simulink model "mainV02_37"  (R2016b)
settings: Solver=FixedStepAuto  StartTime=0.0  StopTime=inf  FixedStep=Ts  MaxStep=0.2  RelTol=1e-2
undefined symbols (not defined in the file): checks, deltae_degrees, deltafl_degrees, deltafr_degrees, deltar_degrees, deltat_1, deltat_2, deltat_3, deltat_4, deltat_5, Earth, F, ft, groundReaction, initialValues, LD, Light, m, MIL, Newton, Raphson, s, sigbuilder_block, Ts, WGS84
libraries: aerolibutil x19, simulink x17, aerolibtransform2 x7, aerolibasang x4, aerolib6dofsys x4, aerolib6dof2 x4, aerolibwind2 x3, aerolibbdyn x3, aerolibconvert2 x3, aerolibconvert x2, vrlib x2, aerolibatmos2 x1
(part 1 of 5)
settings Model: Creator=Uxío  LastModifiedBy=sork9
settings DataIOCC: ReturnWorkspaceOutputs=on  ReturnWorkspaceOutputsName=spidata
settings OptimizationCC: EfficientMapNaN2IntZero=off  SimCompilerOptimization=on
settings DebuggingCC: ReadBeforeWriteMsg=DisableAll  WriteAfterWriteMsg=DisableAll  WriteAfterReadMsg=DisableAll  MultiTaskDSMMsg=none
settings HardwareCC: TargetBitPerPointer=64  TargetBitPerSizeT=64  TargetBitPerPtrDiffT=64  TargetLongLongMode=on  TargetIntDivRoundTo=Zero  TargetEndianess=LittleEndian  TargetWordSize=64  TargetHWDeviceType=MATLAB Host  ProdEqTarget=off
settings ModelReferenceCC: UpdateModelReferenceTargets=IfOutOfDate
settings SFSimCC: SFSimEcho=off
settings CodeAppCC: MaxIdLength=128
settings GRTTargetCC: TargetLangStandard=C89/C90 (ANSI)  CombineOutputUpdateFcns=off  GRTInterface=on
settings ConfigComp: PSAutoStubLUT=on

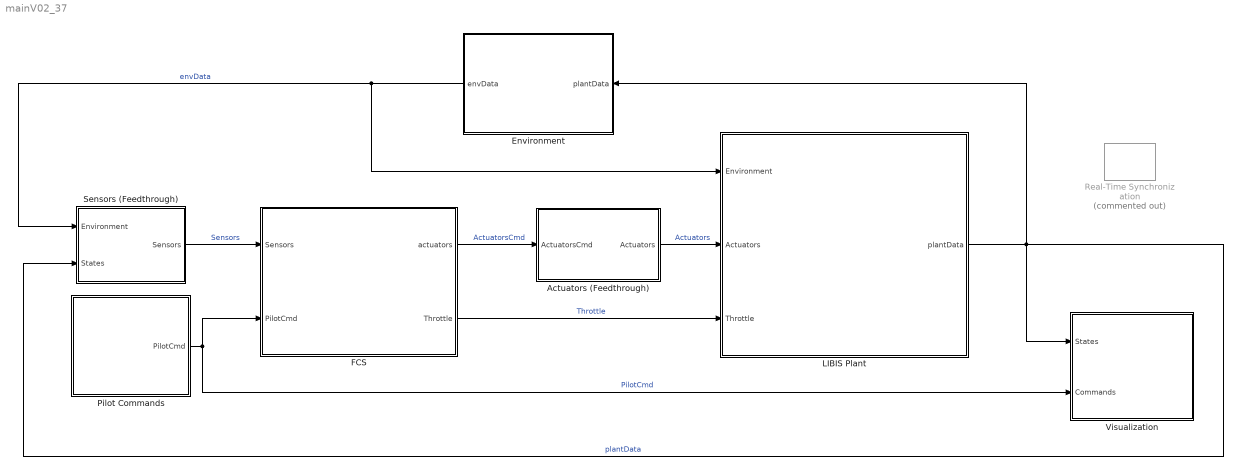
== system mainV02_37 ==
  Actuators (Feedthrough) : Subsystem
  Environment : Subsystem
      mask Display:
      | imageName='Wind.png';
      | currentPath=get_param(bdroot, 'FileName');
      | positions=strfind(currentPath,'\');
      | imagePath=strcat(currentPath(1:positions(end-1)),'graphics\',imageName);
      | image(imagePath);
  FCS : Subsystem
      mask Display:
      | imageName='FCS.png';
      | currentPath=get_param(bdroot, 'FileName');
      | positions=strfind(currentPath,'\');
      | imagePath=strcat(currentPath(1:positions(end-1)),'graphics\',imageName);
      | image(imagePath);
  LIBIS Plant : Subsystem
      mask Display:
      | imageName='LIBIS_Plant.jpg';
      | currentPath=get_param(bdroot, 'FileName');
      | positions=strfind(currentPath,'\');
      | imagePath=strcat(currentPath(1:positions(end-1)),'graphics\',imageName);
      | image(imagePath);
  Pilot Commands : Subsystem  VariantControl=Variants.Command==0
      mask Display:
      | imageName='Pilot.png';
      | currentPath=get_param(bdroot, 'FileName');
      | positions=strfind(currentPath,'\');
      | imagePath=strcat(currentPath(1:positions(end-1)),'graphics\',imageName);
      | image(imagePath);
  Real-Time Synchronization : sldrtlib/Real-Time Synchronization  Commented=on  SampleTime=Ts  MaxMissedTicks=25  ShowMissedTicks=off  YieldWhenWaiting=on
  Sensors (Feedthrough) : Subsystem
  Visualization : Subsystem
  wires:
  FCS/2(Throttle) -> LIBIS Plant/3(Throttle)  "Throttle"
  LIBIS Plant/1(plantData) -> Sensors (Feedthrough)/2(States), Visualization/1(States), Environment/1(plantData)  "plantData"
  Pilot Commands/1(PilotCmd) -> FCS/2(PilotCmd), Visualization/2(Commands)  "PilotCmd"
  Sensors (Feedthrough)/1(Sensors) -> FCS/1(Sensors)  "Sensors"
  Environment/1(envData) -> Sensors (Feedthrough)/1(Environment), LIBIS Plant/1(Environment)  "envData"
  FCS/1(actuators) -> Actuators (Feedthrough)/1(ActuatorsCmd)  "ActuatorsCmd"
  Actuators (Feedthrough)/1(Actuators) -> LIBIS Plant/2(Actuators)  "Actuators"

== system mainV02_37/Actuators (Feedthrough) ==
  ActuatorsCmd : Inport
  Actuators : Outport
  wires:
  ActuatorsCmd/1 -> Actuators/1

== system mainV02_37/Environment ==
  plantData : Inport  OutDataTypeStr=Bus: plantDataBus
  Bus Selector : BusSelector  OutputSignals=LLA.Altitude_m,X_ned,V_ned,Omega_body,CG,DCM_body_earth,LLA.Latitude_deg
  COESA Atmosphere Model : aerolibatmos2/COESA Atmosphere Model  units=Metric (MKS)  spec=1976 COESA-extended U.S. Standard Atmosphere  model=Profile  profile_var=High temperature  profile_percent=1%  profile_alt=5 km (16404 ft)  envelope_var=High temperature  envelope_percent=1%  action=None
  Gravity in Earth Axes : Gain  Gain=[0 0 LD.Inertia.mass]  SaturateOnIntegerOverflow=on  OutDataTypeStr=Inherit: Same as input  ParamDataTypeStr=Inherit: Same as input
  IC : InitialCondition  Value=[0 0 0]
  Math Function : Math  Operator=transpose  SaturateOnIntegerOverflow=on
  Reshape : Reshape
  Reshape1 : Reshape
  Reshape2 : Reshape
  Terrain : Subsystem
  To Body Axes : Product  Multiplication=Matrix(*)  SaturateOnIntegerOverflow=on  InputSameDT=on  OutDataTypeStr=Inherit: Same as first input
  WGS84 Gravity Model : aerolibobsolete/WGS84 Gravity Model  model=WGS84 Taylor Series  units=Metric (MKS)  no_atmos=on  precessing=on  month=February  day=1  year=2000  no_centrifugal=on  action=None
  Wind Models : Subsystem
  envDataBus : BusCreator  Inputs='h_ground','Fground','Mground','windVelocity','windOmega','T','a','P','AirDensity','Fgravity'  OutDataTypeStr=Bus: envDataBus  NonVirtualBus=on
  envData : Outport  OutDataTypeStr=Bus: envDataBus  InitialOutput=0
  wires:
  [Altitude] -> COESA Atmosphere Model/1
  Bus Selector/6 -> To Body Axes/1, Wind Models/3(DCM_be), Terrain/4(DCM_body_earth)  "<DCM_body_earth>"
  Bus Selector/7 -> WGS84 Gravity Model/2  "<Latitude_deg>"
  Bus Selector/3 -> Terrain/2(Ve), Wind Models/1(Ve)  "<V_ned>"
  [Altitude] -> WGS84 Gravity Model/1
  envDataBus/1 -> envData/1  "envData"
  To Body Axes/1 -> Reshape/1  "Fg"
  Wind Models/2(windOmega) -> envDataBus/5  "windOmega"
  Bus Selector/2 -> Terrain/1(Xe)  "<X_ned>"
  WGS84 Gravity Model/1 -> Gravity in Earth Axes/1
  COESA Atmosphere Model/3 -> envDataBus/8  "P"
  COESA Atmosphere Model/2 -> envDataBus/7  "a"
  Wind Models/1(windVelocity) -> envDataBus/4  "windVelocity"
  [Altitude] -> Wind Models/2(Altitude)
  COESA Atmosphere Model/1 -> envDataBus/6  "T"
  COESA Atmosphere Model/4 -> envDataBus/9  "AirDensity"
  Terrain/1(hground) -> envDataBus/1  "h_ground"
  Bus Selector/1 -> [Altitude]  "<Altitude_m>"
  Gravity in Earth Axes/1 -> Math Function/1
  Math Function/1 -> To Body Axes/2
  Reshape/1 -> envDataBus/10  "Fgravity"
  Reshape1/1 -> envDataBus/2  "Fground"
  plantData/1 -> Bus Selector/1
  Bus Selector/5 -> Terrain/5("CG ")  "<CG>"
  Reshape2/1 -> envDataBus/3  "Mground"
  Bus Selector/4 -> Terrain/3("Omega_body ")  "<Omega_body>"
  Terrain/2(Fground) -> IC/1
  Terrain/3(Mground) -> Reshape2/1
  IC/1 -> Reshape1/1

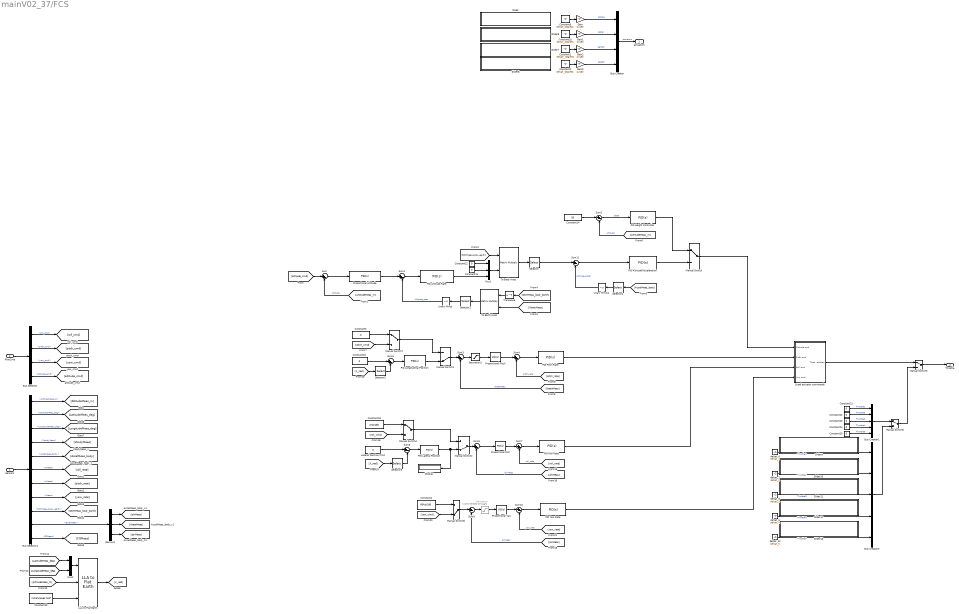
== system mainV02_37/FCS ==
  Sensors : Inport  OutDataTypeStr=Bus: SensorsBus
  PilotCmd : Inport  Port=2  OutDataTypeStr=Bus: CommandBus
  Bus Creator : BusCreator  Inputs=4
  Bus Creator1 : BusCreator  Inputs=5  OutDataTypeStr=Bus: ThrottleBus
  Bus Creator3 : BusCreator  Inputs=5
  Bus Selector : BusSelector  OutputSignals=roll_cmd,pitch_cmd,yaw_cmd,altitude_cmd
  Bus Selector1 : BusSelector  OutputSignals=LLAMeas.AltitudeMeas_m,LLAMeas.LatitudeMeas_deg,LLAMeas.LongitudeMeas_deg,VbodyMeas,AccelMeas_body,OmegaMeas_body.pMeas,OmegaMeas_body.qMeas,OmegaMeas_body.rMeas,DCMMeas_body_earth,EulerMeas,CGMeas
  Constant1 : Constant  Value=deltafr_degrees
  Constant10 : Constant  Value=deltar_degrees
  Constant{3,11..12,16,20..24} (9 alike) : Constant  Value=0
  Constant13 : Constant  Value=initialValues.href
  Constant14 : Constant  Value=50
  Constant18 : Constant  Value=2*pi/180
  Constant2 : Constant  Value=deltafl_degrees
  Constant4 : Constant  Value=60*pi/180
  Constant9 : Constant  Value=deltae_degrees
  Demux3 : Demux  Outputs=3
  Display : Display
  Gain{,1..3} (4 alike) : Gain  Gain=pi/180
  LLA to Flat Earth : aerolibtransform2/LLA to Flat Earth  units=Metric (MKS)  ptype=Earth (WGS84)  F=1/298.257223563  R=6378137  LL0=initialValues.LatLong0  psi=0
  Lateral Position Cmd : Constant  Value=0
  Manual Switch{,3..5,7} (5 alike) : ManualSwitch
  Manual Switch1 : ManualSwitch  CurrentSetting=0
  Manual Switch2 : ManualSwitch  CurrentSetting=0
  Manual Switch6 : ManualSwitch  CurrentSetting=0
  Mux1 : Mux  Inputs=3
  Mux2 : Mux  Inputs=2
  PID Altitude Acceleration : simulink/Continuous/PID Controller  Controller=PID  TimeDomain=Continuous-time  SampleTime=-1  IntegratorMethod=Forward Euler  FilterMethod=Forward Euler  Form=Parallel  UseFilter=on  ControllerParametersSource=internal  P=1  I=1  D=0  N=100  InitialConditionSource=internal  InitialConditionForIntegrator=0  InitialConditionForFilter=0  ExternalReset=none  LimitOutput=on  UpperSaturationLimit=1.5*9.81  LowerSaturationLimit=0.5*9.81  LinearizeAsGain=on  AntiWindupMode=none  Kb=1  TrackingMode=off  Kt=1  PParamMin=[]  PParamMax=[]  IParamMin=[]  IParamMax=[]  DParamMin=[]  DParamMax=[]  NParamMin=[]  NParamMax=[]  KbParamMin=[]  KbParamMax=[]  KtParamMin=[]  KtParamMax=[]  POutMin=[]  POutMax=[]  IOutMin=[]  IOutMax=[]  DOutMin=[]  DOutMax=[]  NOutMin=[]  NOutMax=[]  KbOutMin=[]  KbOutMax=[]  KtOutMin=[]  KtOutMax=[]  IntegratorOutMin=[]  IntegratorOutMax=[]  FilterOutMin=[]  FilterOutMax=[]  SumOutMin=[]  SumOutMax=[]  SumI1OutMin=[]  SumI1OutMax=[]  SumI2OutMin=[]  SumI2OutMax=[]  SumI3OutMin=[]  SumI3OutMax=[]  SumDOutMin=[]  SumDOutMax=[]  SaturationOutMin=[]  SaturationOutMax=[]  IntegratorContinuousStateAttributes=''  IntegratorStateMustResolveToSignalObject=off  IntegratorRTWStateStorageClass=Auto  FilterContinuousStateAttributes=''  FilterStateMustResolveToSignalObject=off  FilterRTWStateStorageClass=Auto  DifferentiatorICPrevScaledInput=0  DifferentiatorOutMin=[]  DifferentiatorOutMax=[]
  PID Altitude Rate : simulink/Continuous/PID Controller  Controller=PID  TimeDomain=Continuous-time  SampleTime=-1  IntegratorMethod=Forward Euler  FilterMethod=Forward Euler  Form=Parallel  UseFilter=on  ControllerParametersSource=internal  P=1  I=1  D=0  N=100  InitialConditionSource=internal  InitialConditionForIntegrator=0  InitialConditionForFilter=0  ExternalReset=none  LimitOutput=on  UpperSaturationLimit=1.5*9.81  LowerSaturationLimit=0.5*9.81  LinearizeAsGain=on  AntiWindupMode=none  Kb=1  TrackingMode=off  Kt=1  PParamMin=[]  PParamMax=[]  IParamMin=[]  IParamMax=[]  DParamMin=[]  DParamMax=[]  NParamMin=[]  NParamMax=[]  KbParamMin=[]  KbParamMax=[]  KtParamMin=[]  KtParamMax=[]  POutMin=[]  POutMax=[]  IOutMin=[]  IOutMax=[]  DOutMin=[]  DOutMax=[]  NOutMin=[]  NOutMax=[]  KbOutMin=[]  KbOutMax=[]  KtOutMin=[]  KtOutMax=[]  IntegratorOutMin=[]  IntegratorOutMax=[]  FilterOutMin=[]  FilterOutMax=[]  SumOutMin=[]  SumOutMax=[]  SumI1OutMin=[]  SumI1OutMax=[]  SumI2OutMin=[]  SumI2OutMax=[]  SumI3OutMin=[]  SumI3OutMax=[]  SumDOutMin=[]  SumDOutMax=[]  SaturationOutMin=[]  SaturationOutMax=[]  IntegratorContinuousStateAttributes=''  IntegratorStateMustResolveToSignalObject=off  IntegratorRTWStateStorageClass=Auto  FilterContinuousStateAttributes=''  FilterStateMustResolveToSignalObject=off  FilterRTWStateStorageClass=Auto  DifferentiatorICPrevScaledInput=0  DifferentiatorOutMin=[]  DifferentiatorOutMax=[]
  PID Height Controller : simulink/Continuous/PID Controller  Controller=PID  TimeDomain=Continuous-time  SampleTime=-1  IntegratorMethod=Forward Euler  FilterMethod=Forward Euler  Form=Parallel  UseFilter=on  ControllerParametersSource=internal  P=0.5  I=0.25  D=0.5  N=100  InitialConditionSource=internal  InitialConditionForIntegrator=0  InitialConditionForFilter=0  ExternalReset=none  LimitOutput=on  UpperSaturationLimit=1  LowerSaturationLimit=0  LinearizeAsGain=on  AntiWindupMode=clamping  Kb=1  TrackingMode=off  Kt=1  PParamMin=[]  PParamMax=[]  IParamMin=[]  IParamMax=[]  DParamMin=[]  DParamMax=[]  NParamMin=[]  NParamMax=[]  KbParamMin=[]  KbParamMax=[]  KtParamMin=[]  KtParamMax=[]  POutMin=[]  POutMax=[]  IOutMin=[]  IOutMax=[]  DOutMin=[]  DOutMax=[]  NOutMin=[]  NOutMax=[]  KbOutMin=[]  KbOutMax=[]  KtOutMin=[]  KtOutMax=[]  IntegratorOutMin=[]  IntegratorOutMax=[]  FilterOutMin=[]  FilterOutMax=[]  SumOutMin=[]  SumOutMax=[]  SumI1OutMin=[]  SumI1OutMax=[]  SumI2OutMin=[]  SumI2OutMax=[]  SumI3OutMin=[]  SumI3OutMax=[]  SumDOutMin=[]  SumDOutMax=[]  SaturationOutMin=[]  SaturationOutMax=[]  IntegratorContinuousStateAttributes=''  IntegratorStateMustResolveToSignalObject=off  IntegratorRTWStateStorageClass=Auto  FilterContinuousStateAttributes=''  FilterStateMustResolveToSignalObject=off  FilterRTWStateStorageClass=Auto  DifferentiatorICPrevScaledInput=0  DifferentiatorOutMin=[]  DifferentiatorOutMax=[]
  PID Lateral Position : simulink/Continuous/PID Controller  Controller=PID  TimeDomain=Continuous-time  SampleTime=-1  IntegratorMethod=Forward Euler  FilterMethod=Forward Euler  Form=Parallel  UseFilter=on  ControllerParametersSource=internal  P=0.1  I=0  D=0.3  N=100  InitialConditionSource=internal  InitialConditionForIntegrator=0  InitialConditionForFilter=0  ExternalReset=none  LimitOutput=on  UpperSaturationLimit=30*pi/180  LowerSaturationLimit=-30*pi/180  LinearizeAsGain=on  AntiWindupMode=none  Kb=1  TrackingMode=off  Kt=1  PParamMin=[]  PParamMax=[]  IParamMin=[]  IParamMax=[]  DParamMin=[]  DParamMax=[]  NParamMin=[]  NParamMax=[]  KbParamMin=[]  KbParamMax=[]  KtParamMin=[]  KtParamMax=[]  POutMin=[]  POutMax=[]  IOutMin=[]  IOutMax=[]  DOutMin=[]  DOutMax=[]  NOutMin=[]  NOutMax=[]  KbOutMin=[]  KbOutMax=[]  KtOutMin=[]  KtOutMax=[]  IntegratorOutMin=[]  IntegratorOutMax=[]  FilterOutMin=[]  FilterOutMax=[]  SumOutMin=[]  SumOutMax=[]  SumI1OutMin=[]  SumI1OutMax=[]  SumI2OutMin=[]  SumI2OutMax=[]  SumI3OutMin=[]  SumI3OutMax=[]  SumDOutMin=[]  SumDOutMax=[]  SaturationOutMin=[]  SaturationOutMax=[]  IntegratorContinuousStateAttributes=''  IntegratorStateMustResolveToSignalObject=off  IntegratorRTWStateStorageClass=Auto  FilterContinuousStateAttributes=''  FilterStateMustResolveToSignalObject=off  FilterRTWStateStorageClass=Auto  DifferentiatorICPrevScaledInput=0  DifferentiatorOutMin=[]  DifferentiatorOutMax=[]
  PID Longitudinal Position : simulink/Continuous/PID Controller  Controller=PID  TimeDomain=Continuous-time  SampleTime=-1  IntegratorMethod=Forward Euler  FilterMethod=Forward Euler  Form=Parallel  UseFilter=on  ControllerParametersSource=internal  P=-0.1  I=0  D=-0.3  N=100  InitialConditionSource=internal  InitialConditionForIntegrator=0  InitialConditionForFilter=0  ExternalReset=none  LimitOutput=on  UpperSaturationLimit=30*pi/180  LowerSaturationLimit=-30*pi/180  LinearizeAsGain=on  AntiWindupMode=none  Kb=1  TrackingMode=off  Kt=1  PParamMin=[]  PParamMax=[]  IParamMin=[]  IParamMax=[]  DParamMin=[]  DParamMax=[]  NParamMin=[]  NParamMax=[]  KbParamMin=[]  KbParamMax=[]  KtParamMin=[]  KtParamMax=[]  POutMin=[]  POutMax=[]  IOutMin=[]  IOutMax=[]  DOutMin=[]  DOutMax=[]  NOutMin=[]  NOutMax=[]  KbOutMin=[]  KbOutMax=[]  KtOutMin=[]  KtOutMax=[]  IntegratorOutMin=[]  IntegratorOutMax=[]  FilterOutMin=[]  FilterOutMax=[]  SumOutMin=[]  SumOutMax=[]  SumI1OutMin=[]  SumI1OutMax=[]  SumI2OutMin=[]  SumI2OutMax=[]  SumI3OutMin=[]  SumI3OutMax=[]  SumDOutMin=[]  SumDOutMax=[]  SaturationOutMin=[]  SaturationOutMax=[]  IntegratorContinuousStateAttributes=''  IntegratorStateMustResolveToSignalObject=off  IntegratorRTWStateStorageClass=Auto  FilterContinuousStateAttributes=''  FilterStateMustResolveToSignalObject=off  FilterRTWStateStorageClass=Auto  DifferentiatorICPrevScaledInput=0  DifferentiatorOutMin=[]  DifferentiatorOutMax=[]
  PID Pitch Rate : simulink/Continuous/PID Controller  Controller=PID  TimeDomain=Continuous-time  SampleTime=-1  IntegratorMethod=Forward Euler  FilterMethod=Forward Euler  Form=Parallel  UseFilter=on  ControllerParametersSource=internal  P=2  I=1  D=0  N=100  InitialConditionSource=internal  InitialConditionForIntegrator=0  InitialConditionForFilter=0  ExternalReset=none  LimitOutput=on  UpperSaturationLimit=0.5  LowerSaturationLimit=-0.5  LinearizeAsGain=on  AntiWindupMode=none  Kb=1  TrackingMode=off  Kt=1  PParamMin=[]  PParamMax=[]  IParamMin=[]  IParamMax=[]  DParamMin=[]  DParamMax=[]  NParamMin=[]  NParamMax=[]  KbParamMin=[]  KbParamMax=[]  KtParamMin=[]  KtParamMax=[]  POutMin=[]  POutMax=[]  IOutMin=[]  IOutMax=[]  DOutMin=[]  DOutMax=[]  NOutMin=[]  NOutMax=[]  KbOutMin=[]  KbOutMax=[]  KtOutMin=[]  KtOutMax=[]  IntegratorOutMin=[]  IntegratorOutMax=[]  FilterOutMin=[]  FilterOutMax=[]  SumOutMin=[]  SumOutMax=[]  SumI1OutMin=[]  SumI1OutMax=[]  SumI2OutMin=[]  SumI2OutMax=[]  SumI3OutMin=[]  SumI3OutMax=[]  SumDOutMin=[]  SumDOutMax=[]  SaturationOutMin=[]  SaturationOutMax=[]  IntegratorContinuousStateAttributes=''  IntegratorStateMustResolveToSignalObject=off  IntegratorRTWStateStorageClass=Auto  FilterContinuousStateAttributes=''  FilterStateMustResolveToSignalObject=off  FilterRTWStateStorageClass=Auto  DifferentiatorICPrevScaledInput=0  DifferentiatorOutMin=[]  DifferentiatorOutMax=[]
  PID Roll Rate : simulink/Continuous/PID Controller  Controller=PID  TimeDomain=Continuous-time  SampleTime=-1  IntegratorMethod=Forward Euler  FilterMethod=Forward Euler  Form=Parallel  UseFilter=on  ControllerParametersSource=internal  P=4  I=0  D=0  N=100  InitialConditionSource=internal  InitialConditionForIntegrator=0  InitialConditionForFilter=0  ExternalReset=none  LimitOutput=on  UpperSaturationLimit=0.5  LowerSaturationLimit=-0.5  LinearizeAsGain=on  AntiWindupMode=none  Kb=1  TrackingMode=off  Kt=1  PParamMin=[]  PParamMax=[]  IParamMin=[]  IParamMax=[]  DParamMin=[]  DParamMax=[]  NParamMin=[]  NParamMax=[]  KbParamMin=[]  KbParamMax=[]  KtParamMin=[]  KtParamMax=[]  POutMin=[]  POutMax=[]  IOutMin=[]  IOutMax=[]  DOutMin=[]  DOutMax=[]  NOutMin=[]  NOutMax=[]  KbOutMin=[]  KbOutMax=[]  KtOutMin=[]  KtOutMax=[]  IntegratorOutMin=[]  IntegratorOutMax=[]  FilterOutMin=[]  FilterOutMax=[]  SumOutMin=[]  SumOutMax=[]  SumI1OutMin=[]  SumI1OutMax=[]  SumI2OutMin=[]  SumI2OutMax=[]  SumI3OutMin=[]  SumI3OutMax=[]  SumDOutMin=[]  SumDOutMax=[]  SaturationOutMin=[]  SaturationOutMax=[]  IntegratorContinuousStateAttributes=''  IntegratorStateMustResolveToSignalObject=off  IntegratorRTWStateStorageClass=Auto  FilterContinuousStateAttributes=''  FilterStateMustResolveToSignalObject=off  FilterRTWStateStorageClass=Auto  DifferentiatorICPrevScaledInput=0  DifferentiatorOutMin=[]  DifferentiatorOutMax=[]
  PID Yaw Rate : simulink/Continuous/PID Controller  Controller=PID  TimeDomain=Continuous-time  SampleTime=-1  IntegratorMethod=Forward Euler  FilterMethod=Forward Euler  Form=Parallel  UseFilter=on  ControllerParametersSource=internal  P=5  I=0  D=0  N=100  InitialConditionSource=internal  InitialConditionForIntegrator=0  InitialConditionForFilter=0  ExternalReset=none  LimitOutput=on  UpperSaturationLimit=0.1  LowerSaturationLimit=-0.1  LinearizeAsGain=on  AntiWindupMode=none  Kb=1  TrackingMode=off  Kt=1  PParamMin=[]  PParamMax=[]  IParamMin=[]  IParamMax=[]  DParamMin=[]  DParamMax=[]  NParamMin=[]  NParamMax=[]  KbParamMin=[]  KbParamMax=[]  KtParamMin=[]  KtParamMax=[]  POutMin=[]  POutMax=[]  IOutMin=[]  IOutMax=[]  DOutMin=[]  DOutMax=[]  NOutMin=[]  NOutMax=[]  KbOutMin=[]  KbOutMax=[]  KtOutMin=[]  KtOutMax=[]  IntegratorOutMin=[]  IntegratorOutMax=[]  FilterOutMin=[]  FilterOutMax=[]  SumOutMin=[]  SumOutMax=[]  SumI1OutMin=[]  SumI1OutMax=[]  SumI2OutMin=[]  SumI2OutMax=[]  SumI3OutMin=[]  SumI3OutMax=[]  SumDOutMin=[]  SumDOutMax=[]  SaturationOutMin=[]  SaturationOutMax=[]  IntegratorContinuousStateAttributes=''  IntegratorStateMustResolveToSignalObject=off  IntegratorRTWStateStorageClass=Auto  FilterContinuousStateAttributes=''  FilterStateMustResolveToSignalObject=off  FilterRTWStateStorageClass=Auto  DifferentiatorICPrevScaledInput=0  DifferentiatorOutMin=[]  DifferentiatorOutMax=[]
  Proportional Altitude : simulink/Continuous/PID Controller  Controller=PID  TimeDomain=Continuous-time  SampleTime=-1  IntegratorMethod=Forward Euler  FilterMethod=Forward Euler  Form=Parallel  UseFilter=on  ControllerParametersSource=internal  P=-1  I=0  D=0  N=100  InitialConditionSource=internal  InitialConditionForIntegrator=0  InitialConditionForFilter=0  ExternalReset=none  LimitOutput=on  UpperSaturationLimit=250  LowerSaturationLimit=-inf  LinearizeAsGain=on  AntiWindupMode=none  Kb=1  TrackingMode=off  Kt=1  PParamMin=[]  PParamMax=[]  IParamMin=[]  IParamMax=[]  DParamMin=[]  DParamMax=[]  NParamMin=[]  NParamMax=[]  KbParamMin=[]  KbParamMax=[]  KtParamMin=[]  KtParamMax=[]  POutMin=[]  POutMax=[]  IOutMin=[]  IOutMax=[]  DOutMin=[]  DOutMax=[]  NOutMin=[]  NOutMax=[]  KbOutMin=[]  KbOutMax=[]  KtOutMin=[]  KtOutMax=[]  IntegratorOutMin=[]  IntegratorOutMax=[]  FilterOutMin=[]  FilterOutMax=[]  SumOutMin=[]  SumOutMax=[]  SumI1OutMin=[]  SumI1OutMax=[]  SumI2OutMin=[]  SumI2OutMax=[]  SumI3OutMin=[]  SumI3OutMax=[]  SumDOutMin=[]  SumDOutMax=[]  SaturationOutMin=[]  SaturationOutMax=[]  IntegratorContinuousStateAttributes=''  IntegratorStateMustResolveToSignalObject=off  IntegratorRTWStateStorageClass=Auto  FilterContinuousStateAttributes=''  FilterStateMustResolveToSignalObject=off  FilterRTWStateStorageClass=Auto  DifferentiatorICPrevScaledInput=0  DifferentiatorOutMin=[]  DifferentiatorOutMax=[]
  Proportional Pitch : simulink/Continuous/PID Controller  Controller=PID  TimeDomain=Continuous-time  SampleTime=-1  IntegratorMethod=Forward Euler  FilterMethod=Forward Euler  Form=Parallel  UseFilter=on  ControllerParametersSource=internal  P=4  I=0  D=0  N=100  InitialConditionSource=internal  InitialConditionForIntegrator=0  InitialConditionForFilter=0  ExternalReset=none  LimitOutput=off  UpperSaturationLimit=inf  LowerSaturationLimit=-inf  LinearizeAsGain=on  AntiWindupMode=none  Kb=1  TrackingMode=off  Kt=1  PParamMin=[]  PParamMax=[]  IParamMin=[]  IParamMax=[]  DParamMin=[]  DParamMax=[]  NParamMin=[]  NParamMax=[]  KbParamMin=[]  KbParamMax=[]  KtParamMin=[]  KtParamMax=[]  POutMin=[]  POutMax=[]  IOutMin=[]  IOutMax=[]  DOutMin=[]  DOutMax=[]  NOutMin=[]  NOutMax=[]  KbOutMin=[]  KbOutMax=[]  KtOutMin=[]  KtOutMax=[]  IntegratorOutMin=[]  IntegratorOutMax=[]  FilterOutMin=[]  FilterOutMax=[]  SumOutMin=[]  SumOutMax=[]  SumI1OutMin=[]  SumI1OutMax=[]  SumI2OutMin=[]  SumI2OutMax=[]  SumI3OutMin=[]  SumI3OutMax=[]  SumDOutMin=[]  SumDOutMax=[]  SaturationOutMin=[]  SaturationOutMax=[]  IntegratorContinuousStateAttributes=''  IntegratorStateMustResolveToSignalObject=off  IntegratorRTWStateStorageClass=Auto  FilterContinuousStateAttributes=''  FilterStateMustResolveToSignalObject=off  FilterRTWStateStorageClass=Auto  DifferentiatorICPrevScaledInput=0  DifferentiatorOutMin=[]  DifferentiatorOutMax=[]
  Proportional Roll : simulink/Continuous/PID Controller  Controller=PID  TimeDomain=Continuous-time  SampleTime=-1  IntegratorMethod=Forward Euler  FilterMethod=Forward Euler  Form=Parallel  UseFilter=on  ControllerParametersSource=internal  P=1  I=0  D=0  N=100  InitialConditionSource=internal  InitialConditionForIntegrator=0  InitialConditionForFilter=0  ExternalReset=none  LimitOutput=off  UpperSaturationLimit=inf  LowerSaturationLimit=-inf  LinearizeAsGain=on  AntiWindupMode=none  Kb=1  TrackingMode=off  Kt=1  PParamMin=[]  PParamMax=[]  IParamMin=[]  IParamMax=[]  DParamMin=[]  DParamMax=[]  NParamMin=[]  NParamMax=[]  KbParamMin=[]  KbParamMax=[]  KtParamMin=[]  KtParamMax=[]  POutMin=[]  POutMax=[]  IOutMin=[]  IOutMax=[]  DOutMin=[]  DOutMax=[]  NOutMin=[]  NOutMax=[]  KbOutMin=[]  KbOutMax=[]  KtOutMin=[]  KtOutMax=[]  IntegratorOutMin=[]  IntegratorOutMax=[]  FilterOutMin=[]  FilterOutMax=[]  SumOutMin=[]  SumOutMax=[]  SumI1OutMin=[]  SumI1OutMax=[]  SumI2OutMin=[]  SumI2OutMax=[]  SumI3OutMin=[]  SumI3OutMax=[]  SumDOutMin=[]  SumDOutMax=[]  SaturationOutMin=[]  SaturationOutMax=[]  IntegratorContinuousStateAttributes=''  IntegratorStateMustResolveToSignalObject=off  IntegratorRTWStateStorageClass=Auto  FilterContinuousStateAttributes=''  FilterStateMustResolveToSignalObject=off  FilterRTWStateStorageClass=Auto  DifferentiatorICPrevScaledInput=0  DifferentiatorOutMin=[]  DifferentiatorOutMax=[]
  Proportional Yaw : simulink/Continuous/PID Controller  Controller=PID  TimeDomain=Continuous-time  SampleTime=-1  IntegratorMethod=Forward Euler  FilterMethod=Forward Euler  Form=Parallel  UseFilter=on  ControllerParametersSource=internal  P=1  I=0  D=0  N=100  InitialConditionSource=internal  InitialConditionForIntegrator=0  InitialConditionForFilter=0  ExternalReset=none  LimitOutput=off  UpperSaturationLimit=30*pi/180  LowerSaturationLimit=-30*pi/180  LinearizeAsGain=on  AntiWindupMode=none  Kb=1  TrackingMode=off  Kt=1  PParamMin=[]  PParamMax=[]  IParamMin=[]  IParamMax=[]  DParamMin=[]  DParamMax=[]  NParamMin=[]  NParamMax=[]  KbParamMin=[]  KbParamMax=[]  KtParamMin=[]  KtParamMax=[]  POutMin=[]  POutMax=[]  IOutMin=[]  IOutMax=[]  DOutMin=[]  DOutMax=[]  NOutMin=[]  NOutMax=[]  KbOutMin=[]  KbOutMax=[]  KtOutMin=[]  KtOutMax=[]  IntegratorOutMin=[]  IntegratorOutMax=[]  FilterOutMin=[]  FilterOutMax=[]  SumOutMin=[]  SumOutMax=[]  SumI1OutMin=[]  SumI1OutMax=[]  SumI2OutMin=[]  SumI2OutMax=[]  SumI3OutMin=[]  SumI3OutMax=[]  SumDOutMin=[]  SumDOutMax=[]  SaturationOutMin=[]  SaturationOutMax=[]  IntegratorContinuousStateAttributes=''  IntegratorStateMustResolveToSignalObject=off  IntegratorRTWStateStorageClass=Auto  FilterContinuousStateAttributes=''  FilterStateMustResolveToSignalObject=off  FilterRTWStateStorageClass=Auto  DifferentiatorICPrevScaledInput=0  DifferentiatorOutMin=[]  DifferentiatorOutMax=[]
  Quad actuator commands : Subsystem
  Saturation : Saturate  Commented=through  UpperLimit=30*pi/180  LowerLimit=-30*pi/180
  Saturation1 : Saturate  UpperLimit=30*pi/180  LowerLimit=-30*pi/180
  Selector : Selector  InputPortWidth=3  IndexOptions=Index vector (dialog)  Indices=[ 3]  OutputSizes=1
  Selector1 : Selector  InputPortWidth=3  IndexOptions=Index vector (dialog)  Indices=[ 3]  OutputSizes=1
  Selector2 : Selector  InputPortWidth=3  IndexOptions=Index vector (dialog)  Indices=1  OutputSizes=1
  Selector3 : Selector  InputPortWidth=3  IndexOptions=Index vector (dialog)  Indices=2  OutputSizes=1
  Selector4 : Selector  InputPortWidth=3  IndexOptions=Index vector (dialog)  Indices=[3]  OutputSizes=1
  Slider : Subsystem  DialogController=hmiCreateDDGDialog  IsWebBlock=on  mask(MWDashboardBlock){webBlockId=6273dd38-214f-4c77-9b1a-24b6ec7057c4, webBlockType=slider, ShowInLibBrowser=on, ShowInitialText=on, HMISrcModelName=mainV02_33}
      mask prompts: webBlockId "WebBlock Id"; webBlockType "WebBlock Type"; HMISrcModelName "Source Model"
      mask help: SimulinkHMI:dialogs:SliderDialogDesc
      mask Help: helpview([docroot '/mapfiles/simulink.map'], 'hmi_slider')
      mask Display:
      | if strcmp(get_param(bdroot(gcb),'BlockDiagramType'), 'library')
      |     image([(matlabroot) '/toolbox/simulink/hmi/icons/Slider.png']);
      | end
  Slider10 : Subsystem  DialogController=hmiCreateDDGDialog  IsWebBlock=on  mask(MWDashboardBlock){webBlockId=00630764-615e-4f17-a60f-cb6c0864fa70, webBlockType=slider, ShowInLibBrowser=on, ShowInitialText=on, HMISrcModelName=mainV02_33}
      mask prompts: webBlockId "WebBlock Id"; webBlockType "WebBlock Type"; HMISrcModelName "Source Model"
      mask help: SimulinkHMI:dialogs:SliderDialogDesc
      mask Help: helpview([docroot '/mapfiles/simulink.map'], 'hmi_slider')
      mask Display:
      | if strcmp(get_param(bdroot(gcb),'BlockDiagramType'), 'library')
      |     image([(matlabroot) '/toolbox/simulink/hmi/icons/Slider.png']);
      | end
  Slider11 : Subsystem  DialogController=hmiCreateDDGDialog  IsWebBlock=on  mask(MWDashboardBlock){webBlockId=0dfd5fba-0907-4f81-8c64-99d41af2b5a5, webBlockType=slider, ShowInLibBrowser=on, ShowInitialText=on, HMISrcModelName=mainV02_33}
      mask prompts: webBlockId "WebBlock Id"; webBlockType "WebBlock Type"; HMISrcModelName "Source Model"
      mask help: SimulinkHMI:dialogs:SliderDialogDesc
      mask Help: helpview([docroot '/mapfiles/simulink.map'], 'hmi_slider')
      mask Display:
      | if strcmp(get_param(bdroot(gcb),'BlockDiagramType'), 'library')
      |     image([(matlabroot) '/toolbox/simulink/hmi/icons/Slider.png']);
      | end
  Slider12 : Subsystem  DialogController=hmiCreateDDGDialog  IsWebBlock=on  mask(MWDashboardBlock){webBlockId=467649b1-ad24-470a-ba7c-8391d4687733, webBlockType=slider, ShowInLibBrowser=on, ShowInitialText=on, HMISrcModelName=mainV02_33}
      mask prompts: webBlockId "WebBlock Id"; webBlockType "WebBlock Type"; HMISrcModelName "Source Model"
      mask help: SimulinkHMI:dialogs:SliderDialogDesc
      mask Help: helpview([docroot '/mapfiles/simulink.map'], 'hmi_slider')
      mask Display:
      | if strcmp(get_param(bdroot(gcb),'BlockDiagramType'), 'library')
      |     image([(matlabroot) '/toolbox/simulink/hmi/icons/Slider.png']);
      | end
  Slider13 : Subsystem  DialogController=hmiCreateDDGDialog  IsWebBlock=on  mask(MWDashboardBlock){webBlockId=6807b92d-ffd5-4861-aff5-f6e71f5481f5, webBlockType=slider, ShowInLibBrowser=on, ShowInitialText=on, HMISrcModelName=mainV02_33}
      mask prompts: webBlockId "WebBlock Id"; webBlockType "WebBlock Type"; HMISrcModelName "Source Model"
      mask help: SimulinkHMI:dialogs:SliderDialogDesc
      mask Help: helpview([docroot '/mapfiles/simulink.map'], 'hmi_slider')
      mask Display:
      | if strcmp(get_param(bdroot(gcb),'BlockDiagramType'), 'library')
      |     image([(matlabroot) '/toolbox/simulink/hmi/icons/Slider.png']);
      | end
  Slider6 : Subsystem  DialogController=hmiCreateDDGDialog  IsWebBlock=on  mask(MWDashboardBlock){webBlockId=3d9f47b7-f15d-42be-b3f0-4bf7c2d4a508, webBlockType=slider, ShowInLibBrowser=on, ShowInitialText=on, HMISrcModelName=mainV02_33}
      mask prompts: webBlockId "WebBlock Id"; webBlockType "WebBlock Type"; HMISrcModelName "Source Model"
      mask help: SimulinkHMI:dialogs:SliderDialogDesc
      mask Help: helpview([docroot '/mapfiles/simulink.map'], 'hmi_slider')
      mask Display:
      | if strcmp(get_param(bdroot(gcb),'BlockDiagramType'), 'library')
      |     image([(matlabroot) '/toolbox/simulink/hmi/icons/Slider.png']);
      | end
  Slider7 : Subsystem  DialogController=hmiCreateDDGDialog  IsWebBlock=on  mask(MWDashboardBlock){webBlockId=8e5c7658-11f4-4f70-8154-234cc52576e8, webBlockType=slider, ShowInLibBrowser=on, ShowInitialText=on, HMISrcModelName=mainV02_33}
      mask prompts: webBlockId "WebBlock Id"; webBlockType "WebBlock Type"; HMISrcModelName "Source Model"
      mask help: SimulinkHMI:dialogs:SliderDialogDesc
      mask Help: helpview([docroot '/mapfiles/simulink.map'], 'hmi_slider')
      mask Display:
      | if strcmp(get_param(bdroot(gcb),'BlockDiagramType'), 'library')
      |     image([(matlabroot) '/toolbox/simulink/hmi/icons/Slider.png']);
      | end
  Slider8 : Subsystem  DialogController=hmiCreateDDGDialog  IsWebBlock=on  mask(MWDashboardBlock){webBlockId=fd4f6454-3dcd-4a0d-9f3e-71aa520b8d15, webBlockType=slider, ShowInLibBrowser=on, ShowInitialText=on, HMISrcModelName=mainV02_33}
      mask prompts: webBlockId "WebBlock Id"; webBlockType "WebBlock Type"; HMISrcModelName "Source Model"
      mask help: SimulinkHMI:dialogs:SliderDialogDesc
      mask Help: helpview([docroot '/mapfiles/simulink.map'], 'hmi_slider')
      mask Display:
      | if strcmp(get_param(bdroot(gcb),'BlockDiagramType'), 'library')
      |     image([(matlabroot) '/toolbox/simulink/hmi/icons/Slider.png']);
      | end
  Slider9 : Subsystem  DialogController=hmiCreateDDGDialog  IsWebBlock=on  mask(MWDashboardBlock){webBlockId=8d33ebc5-b5df-45a1-b533-c20d4efea2ab, webBlockType=slider, ShowInLibBrowser=on, ShowInitialText=on, HMISrcModelName=mainV02_33}
      mask prompts: webBlockId "WebBlock Id"; webBlockType "WebBlock Type"; HMISrcModelName "Source Model"
      mask help: SimulinkHMI:dialogs:SliderDialogDesc
      mask Help: helpview([docroot '/mapfiles/simulink.map'], 'hmi_slider')
      mask Display:
      | if strcmp(get_param(bdroot(gcb),'BlockDiagramType'), 'library')
      |     image([(matlabroot) '/toolbox/simulink/hmi/icons/Slider.png']);
      | end
  Sum{,1..11} (12 alike) : Sum  Inputs=|+-
  To Body Axes : Product  Multiplication=Matrix(*)  SaturateOnIntegerOverflow=on  InputSameDT=on  OutDataTypeStr=Inherit: Same as first input
  To Earth Axes : Product  Multiplication=Matrix(*)  SaturateOnIntegerOverflow=on  InputSameDT=on  OutDataTypeStr=Inherit: Same as first input
  Transpose : Math  Operator=transpose  SaturateOnIntegerOverflow=on
  Unary Minus : UnaryMinus
  Unary Minus1 : UnaryMinus
  deltat_10 : Constant  Value=deltat_5
  deltat_6 : Constant  Value=deltat_1
  deltat_7 : Constant  Value=deltat_2
  deltat_8 : Constant  Value=deltat_3
  deltat_9 : Constant  Value=deltat_4
  actuators : Outport
  Throttle : Outport  Port=2  OutDataTypeStr=Bus: ThrottleBus
  wires:
  PilotCmd/1 -> Bus Selector/1
  Sensors/1 -> Bus Selector1/1
  Bus Creator/1 -> actuators/1  "actuators"
  Gain1/1 -> Bus Creator/2  "deltar"
  Gain2/1 -> Bus Creator/3  "deltafr"
  Gain3/1 -> Bus Creator/4  "deltafl"
  Gain/1 -> Bus Creator/1  "deltae"
  Constant10/1 -> Gain1/1
  Constant1/1 -> Gain2/1
  Constant2/1 -> Gain3/1
  Bus Selector1/1 -> [AltitudeMeas_m]  "<AltitudeMeas_m>"
  Bus Selector/1 -> [roll_cmd]  "<roll_cmd>"
  Bus Selector/2 -> [pitch_cmd]  "<pitch_cmd>"
  Bus Selector/3 -> [yaw_cmd]  "<yaw_cmd>"
  Bus Selector/4 -> [altitude_cmd]  "<altitude_cmd>"
  Bus Selector1/6 -> [roll_rate]  "<pMeas>"
  Bus Selector1/7 -> [pitch_rate]  "<qMeas>"
  Bus Selector1/8 -> [yaw_rate]  "<rMeas>"
  [altitude_cmd] -> Sum/1
  [AltitudeMeas_m] -> Sum/2  "Altitude"
  Sum/1 -> Proportional Altitude/1
  Proportional Altitude/1 -> Sum1/1
  Sum1/1 -> PID Altitude Rate/1
  Constant11/1 -> Mux1/2
  Constant12/1 -> Mux1/1
  Mux1/1 -> To Body Axes/2
  PID Altitude Rate/1 -> Mux1/3
  [DCMMeas_body_earth] -> To Body Axes/1
  To Body Axes/1 -> Selector/1
  Bus Selector1/9 -> [DCMMeas_body_earth]  "<DCMMeas_body_earth>"
  [DCMMeas_body_earth] -> Transpose/1
  Transpose/1 -> To Earth Axes/1
  To Earth Axes/1 -> Selector1/1
  Selector1/1 -> Unary Minus/1
  Sum2/1 -> PID Height Controller/1  "delta"
  Unary Minus/1 -> Sum1/2  "Altitude_rate"
  Constant14/1 -> Sum2/1
  Unary Minus1/1 -> Sum11/2  "Altitude_accel"
  [AltitudeMeas_m] -> Sum2/2  "Altitude"
  Bus Selector1/10 -> Demux3/1  "<EulerMeas>"
  Demux3/1 -> [phiMeas]
  Demux3/2 -> [thetaMeas]
  Demux3/3 -> [psiMeas]
  [thetaMeas] -> Sum3/2  "thetaMeas"
  Sum3/1 -> Saturation1/1
  [pitch_rate] -> Sum4/2  "pitch_rate"
  Proportional Pitch/1 -> Sum4/1
  Sum4/1 -> PID Pitch Rate/1
  PID Pitch Rate/1 -> Quad actuator commands/2(Pitch cmd)
  Constant9/1 -> Gain/1
  [pitch_cmd] -> Manual Switch7/2
  Bus Selector1/11 -> [CGMeas]  "<CGMeas>"
  Bus Selector1/2 -> [LatitudeMeas_deg]  "<LatitudeMeas_deg>"
  Bus Selector1/3 -> [LongitudeMeas_deg]  "<LongitudeMeas_deg>"
  Constant13/1 -> LLA to Flat Earth/3
  [AltitudeMeas_m] -> LLA to Flat Earth/2
  [LatitudeMeas_deg] -> Mux2/1
  [LongitudeMeas_deg] -> Mux2/2
  Mux2/1 -> LLA to Flat Earth/1
  LLA to Flat Earth/1 -> [X_ned]
  [X_ned] -> Selector2/1
  Selector2/1 -> Sum5/2
  PID Longitudinal Position/1 -> Manual Switch1/2
  Manual Switch1/1 -> Sum3/1
  [phiMeas] -> Sum6/2  "phiMeas"
  Sum6/1 -> Proportional Roll/1
  [roll_rate] -> Sum7/2  "roll_rate"
  Proportional Roll/1 -> Sum7/1
  Sum7/1 -> PID Roll Rate/1
  PID Roll Rate/1 -> Quad actuator commands/3(Roll cmd)
  [X_ned] -> Selector3/1
  Selector3/1 -> Sum8/2
  Lateral Position Cmd/1 -> Sum8/1
  Sum8/1 -> PID Lateral Position/1
  PID Lateral Position/1 -> Manual Switch2/2, Display/1
  Manual Switch2/1 -> Sum6/1
  Manual Switch4/1 -> Manual Switch2/1
  Constant21/1 -> Bus Creator1/1  "Throttle1"
  Constant23/1 -> Bus Creator1/3  "Throttle3"
  Constant22/1 -> Bus Creator1/2  "Throttle2"
  Constant24/1 -> Bus Creator1/4  "Throttle4"
  Constant20/1 -> Bus Creator1/5  "Throttle5"
  Manual Switch3/1 -> Throttle/1
  Quad actuator commands/1(Throttle_Quadrotor) -> Manual Switch3/1
  deltat_6/1 -> Bus Creator3/1  "Throttle1"
  deltat_8/1 -> Bus Creator3/3  "Throttle3"
  deltat_7/1 -> Bus Creator3/2  "Throttle2"
  deltat_9/1 -> Bus Creator3/4  "Throttle4"
  deltat_10/1 -> Bus Creator3/5  "Throttle5"
  Bus Creator1/1 -> Manual Switch5/1
  Bus Creator3/1 -> Manual Switch5/2
  Manual Switch5/1 -> Manual Switch3/2
  [psiMeas] -> Sum9/2  "psiMeas"
  Sum9/1 -> Saturation/1
  [yaw_rate] -> Sum10/2  "yaw_rate"
  Proportional Yaw/1 -> Sum10/1
  Sum10/1 -> PID Yaw Rate/1
  [yaw_cmd] -> Manual Switch6/2
  PID Yaw Rate/1 -> Quad actuator commands/4(Yaw cmd)
  Sum5/1 -> PID Longitudinal Position/1
  Constant16/1 -> Sum5/1
  Constant4/1 -> Manual Switch6/1
  Manual Switch6/1 -> Sum9/1
  Saturation/1 -> Proportional Yaw/1
  Saturation1/1 -> Proportional Pitch/1
  Constant18/1 -> Manual Switch4/1
  [roll_cmd] -> Manual Switch4/2
  Constant3/1 -> Manual Switch7/1
  Manual Switch7/1 -> Manual Switch1/1
  Bus Selector1/4 -> [VbodyMeas]  "<VbodyMeas>"
  [VbodyMeas] -> To Earth Axes/2
  Bus Selector1/5 -> [AccelMeas_body]  "<AccelMeas_body>"
  Selector4/1 -> Unary Minus1/1
  [AccelMeas_body] -> Selector4/1
  Sum11/1 -> PID Altitude Acceleration/1
  Selector/1 -> Sum11/1
  PID Altitude Acceleration/1 -> Manual Switch/2
  PID Height Controller/1 -> Manual Switch/1
  Manual Switch/1 -> Quad actuator commands/1(Altitude cmd)

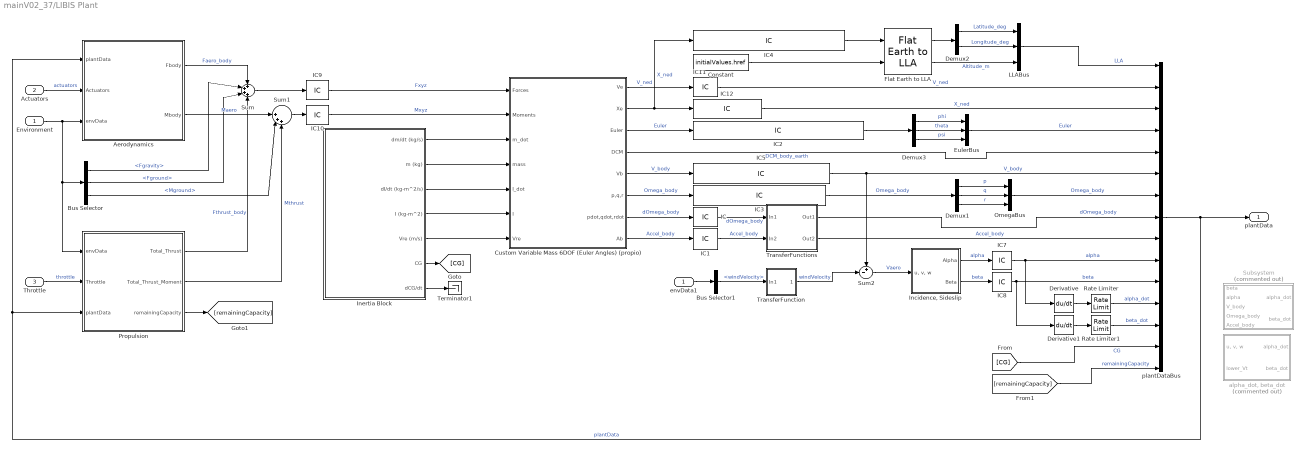
== system mainV02_37/LIBIS Plant ==
  Environment : Inport  OutDataTypeStr=Bus: envDataBus
  Actuators : Inport  Port=2
  Throttle : Inport  Port=3  OutDataTypeStr=Bus: ThrottleBus
  Aerodynamics : Subsystem
  Bus Selector : BusSelector  OutputSignals=Fgravity,Fground,Mground
  Bus Selector1 : BusSelector  OutputSignals=windVelocity
  Constant : Constant  Value=initialValues.href
  Custom Variable Mass 6DOF (Euler Angles) (propio) : Subsystem  mask(6DOF EoM (Body Axis)){units=Metric (MKS), mtype=Custom Variable, rep=Euler Angles, xme_0=[initialValues.Xe0 initialValues.Ye0 initialValues.Ze0], Vm_0=[initialValues.u0 initialValues.v0 initialValues.w0], eul_0=[initialValues.roll0 initialValues.pitch0 initialValues.yaw0], pm_0=[initialValues.p0 initialValues.q0 initialValues.r0], mass_0=1.0, mass_e=0.5, mass_f=2.0, inertia=eye(3), inertia_e=eye(3), inertia_f=2*eye(3), k_quat=1.0, vre_flag=on}
      mask prompts: units "aeroblks:aeroblk6dofbody:block6DOFEoMBodyAxisParamUnits"; mtype "aeroblks:aeroblk6dofbody:block6DOFEoMBodyAxisParamMasstype"; rep "aeroblks:aeroblk6dofbody:block6DOFEoMBodyAxisParamRepresentation"; xme_0 "aeroblks:aeroblk6dofbody:block6DOFEoMBodyAxisParamInitialpositionininertialaxesXeYeZe"; Vm_0 "aeroblks:aeroblk6dofbody:block6DOFEoMBodyAxisParamInitialvelocityinbodyaxesUvw"; eul_0 "aeroblks:aeroblk6dofbody:block6DOFEoMBodyAxisParamInitialEulerorientationrollpitchyaw"; pm_0 "aeroblks:aeroblk6dofbody:block6DOFEoMBodyAxisParamInitialbodyrotationratespqr"; mass_0 "aeroblks:aeroblk6dofbody:block6DOFEoMBodyAxisParamInitialmass"; mass_e "aeroblks:aeroblk6dofbody:block6DOFEoMBodyAxisParamEmptymass"; mass_f "aeroblks:aeroblk6dofbody:block6DOFEoMBodyAxisParamFullmass"; inertia "aeroblks:aeroblk6dofbody:block6DOFEoMBodyAxisParamInertia"; inertia_e "aeroblks:aeroblk6dofbody:block6DOFEoMBodyAxisParamEmptyinertiamatrix"; inertia_f "aeroblks:aeroblk6dofbody:block6DOFEoMBodyAxisParamFullinertiamatrix"; k_quat "aeroblks:aeroblk6dofbody:block6DOFEoMBodyAxisParamGainforquaternionnormalization"; vre_flag "aeroblks:aeroblk6dofbody:block6DOFEoMBodyAxisParamIncludemassflowrelativevelocity"
      mask help: aeroblks:aeroblk6dofbody:block6DOFEoMBodyAxisDesc
      mask init:
      | ports=aeroicon('aeroblk6dofbody','icon');
      mask Help: eval('asbhelp(''custom_variable_mass_sixdof_euler_angles'')');
      mask TypeOptions units: aeroblks:aeroblk6dofbody:block6DOFEoMBodyAxisParamComboMetricMKS | aeroblks:aeroblk6dofbody:block6DOFEoMBodyAxisParamComboEnglishVelocityinfts | aeroblks:aeroblk6dofbody:block6DOFEoMBodyAxisParamComboEnglishVelocityinkts
      mask TypeOptions mtype: aeroblks:aeroblk6dofbody:block6DOFEoMBodyAxisParamComboFixed | aeroblks:aeroblk6dofbody:block6DOFEoMBodyAxisParamComboSimpleVariable | aeroblks:aeroblk6dofbody:block6DOFEoMBodyAxisParamComboCustomVariable
      mask Callback mtype: aeroicon('aeroblk6dofbody');
      mask TypeOptions rep: aeroblks:aeroblk6dofbody:block6DOFEoMBodyAxisParamComboEulerAngles | aeroblks:aeroblk6dofbody:block6DOFEoMBodyAxisParamComboQuaternion
      mask Callback rep: aeroicon('aeroblk6dofbody');
      mask Display:
      | port_label(ports(1).type,ports(1).port,ports(1).txt,'texmode','on');
      | port_label(ports(2).type,ports(2).port,ports(2).txt,'texmode','on');
      | port_label(ports(3).type,ports(3).port,ports(3).txt,'texmode','on');
      | port_label(ports(4).type,ports(4).port,ports(4).txt,'texmode','on');
      | port_label(ports(5).type,ports(5).port,ports(5).txt,'texmode','on');
      | port_label(ports(6).type,ports(6).port,ports(6).txt,'texmode','on');
      | port_label(ports(7).type,ports(7).port,ports(7).txt,'texmode','on');
      | port_label(ports(8).type,ports(8).port,ports(8).txt,'texmode','on');
      | port_label(ports(9).type,ports(9).port,ports(9).txt,'texmode','on');
      | port_label(ports(10).type,ports(10).port,ports(10).txt,'texmode','on');
      | port_label(ports(11).type,ports(11).port,ports(11).txt,'texmode','on');
      | port_label(ports(12).type,ports(12).port,ports(12).txt,'texmode','on');
      | port_label(ports(13).type,ports(13).port,ports(13).txt,'texmode','on');
      | port_label(ports(14).type,ports(14).port,ports(14).txt,'texmode','on');
      | port_label(ports(15).type,ports(15).port,ports(15).txt,'texmode','on');
      | port_label(ports(16).type,ports(16).port,ports(16).txt,'texmode','on');
      | [x y xp yp highstr lowstr maxy miny]=aeroimage('sixdofbody',gcbh);
      | text(0.5,maxy+0.065,highstr{:},'horizontalAlignment','center')
      | text(0.5,miny-0.06,lowstr{:},'horizontalAlignment','center')
      | plot(x,y);
      | patch(xp, yp);
  Demux1 : Demux  Outputs=3
  Demux2 : Demux  Outputs=2
  Demux3 : Demux  Outputs=3
  Derivative : Derivative
  Derivative1 : Derivative
  EulerBus : BusCreator  Inputs='phi','theta','psi'  OutDataTypeStr=Bus: EulerBus  NonVirtualBus=on
  Flat Earth to LLA : aerolibtransform2/Flat Earth to LLA  units=Metric (MKS)  ptype=Earth (WGS84)  F=1/298.257223563  R=6378137  LL0=initialValues.LatLong0  psi=initialValues.heading0
  IC{,1,9..11} (5 alike) : InitialCondition  Value=[0 0 0]
  IC12 : InitialCondition  Value=[0 0 -initialValues.href]
  IC2 : InitialCondition  Value=[initialValues.roll0, initialValues.pitch0, initialValues.yaw0]
  IC3 : InitialCondition  Value=[initialValues.p0 initialValues.q0 initialValues.r0]
  IC4 : InitialCondition  Value=[initialValues.Xe0 initialValues.Ye0 initialValues.Ze0]
  IC5 : InitialCondition  Value=[initialValues.u0 initialValues.v0 initialValues.w0]
  IC7 : InitialCondition  Value=0
  IC8 : InitialCondition  Value=0
  "Incidence, Sideslip" : Subsystem
  Inertia Block : Subsystem
      mask Display:
      | imageName='Moment_of_inertia.png';
      | currentPath=get_param(bdroot, 'FileName');
      | positions=strfind(currentPath,'\');
      | imagePath=strcat(currentPath(1:positions(end-1)),'graphics\',imageName);
      | image(imagePath);
  LLABus : BusCreator  Inputs='Latitude_deg','Longitude_deg','Altitude_m'  OutDataTypeStr=Bus: LLABus  NonVirtualBus=on
  OmegaBus : BusCreator  Inputs='p','q','r'  OutDataTypeStr=Bus: OmegaBus  NonVirtualBus=on
  Propulsion : Subsystem
  Rate Limiter : RateLimiter  RisingSlewLimit=100  FallingSlewLimit=-100  SampleTimeMode=inherited
  Rate Limiter1 : RateLimiter  RisingSlewLimit=100  FallingSlewLimit=-100  SampleTimeMode=inherited
  Subsystem : Subsystem  Commented=on
  Sum : Sum  Inputs=++++
  Sum1 : Sum  Inputs=||+++
  Sum2 : Sum  Inputs=+-|
  Terminator1 : Terminator
  TransferFunction : Subsystem
  TransferFunctions : Subsystem
  "alpha_dot, beta_dot" : Subsystem  Commented=on
  envData1 : InportShadow  OutDataTypeStr=Bus: envDataBus
  plantDataBus : BusCreator  Inputs='LLA','V_ned','X_ned','Euler','DCM_body_earth','V_body','Omega_body','dOmega_body','Accel_body','alpha','beta','alpha_dot','beta_dot','CG','remainingCapacity'  OutDataTypeStr=Bus: plantDataBus  NonVirtualBus=on
  plantData : Outport  OutDataTypeStr=Bus: plantDataBus
  wires:
  Inertia Block/4(I (kg-m^2)) -> Custom Variable Mass 6DOF (Euler Angles) (propio)/6(I)
  plantDataBus/1 -> Propulsion/3(plantData), Aerodynamics/1(plantData), plantData/1  "plantData"
  Flat Earth to LLA/2 -> LLABus/3  "Altitude_m"
  Custom Variable Mass 6DOF (Euler Angles) (propio)/2(Xe) -> IC12/1, IC4/1  "X_ned"
  Custom Variable Mass 6DOF (Euler Angles) (propio)/3(Euler) -> IC2/1  "Euler"
  EulerBus/1 -> plantDataBus/4  "Euler"
  Flat Earth to LLA/1 -> Demux2/1
  Demux2/1 -> LLABus/1  "Latitude_deg"
  Inertia Block/2(m (kg)) -> Custom Variable Mass 6DOF (Euler Angles) (propio)/4(mass)
  Inertia Block/5(Vre (m/s)) -> Custom Variable Mass 6DOF (Euler Angles) (propio)/7(Vre)
  Custom Variable Mass 6DOF (Euler Angles) (propio)/5(Vb) -> IC5/1  "V_body"
  Inertia Block/7(dCG/dt) -> Terminator1/1
  [CG] -> plantDataBus/14  "CG"
  Custom Variable Mass 6DOF (Euler Angles) (propio)/4(DCM) -> plantDataBus/5  "DCM_body_earth"
  Inertia Block/3(dI/dt (kg-m^2/s)) -> Custom Variable Mass 6DOF (Euler Angles) (propio)/5(I_dot)
  LLABus/1 -> plantDataBus/1  "LLA"
  "Incidence, Sideslip"/1(Alpha) -> IC7/1  "alpha"
  Demux3/1 -> EulerBus/1  "phi"
  Demux3/3 -> EulerBus/3  "psi"
  Inertia Block/6(CG) -> [CG]
  Inertia Block/1(dm/dt (kg/s)) -> Custom Variable Mass 6DOF (Euler Angles) (propio)/3(m_dot)
  Constant/1 -> Flat Earth to LLA/2
  Demux2/2 -> LLABus/2  "Longitude_deg"
  "Incidence, Sideslip"/2(Beta) -> IC8/1  "beta"
  Demux3/2 -> EulerBus/2  "theta"
  Custom Variable Mass 6DOF (Euler Angles) (propio)/1(Ve) -> IC11/1  "V_ned"
  OmegaBus/1 -> plantDataBus/7  "Omega_body"
  Custom Variable Mass 6DOF (Euler Angles) (propio)/6(p,q,r) -> IC3/1  "Omega_body"
  Demux1/2 -> OmegaBus/2  "q"
  Demux1/1 -> OmegaBus/1  "p"
  Demux1/3 -> OmegaBus/3  "r"
  Actuators/1 -> Aerodynamics/2(Actuators)  "actuators"
  Throttle/1 -> Propulsion/2(Throttle)  "throttle"
  Propulsion/3(remainingCapacity) -> [remainingCapacity]
  [remainingCapacity] -> plantDataBus/15  "remainingCapacity"
  Propulsion/1(Total_Thrust) -> Sum/4  "Fthrust_body"
  Environment/1 -> Propulsion/1(envData), Bus Selector/1, Aerodynamics/3(envData)
  IC4/1 -> Flat Earth to LLA/1
  IC5/1 -> plantDataBus/6, Sum2/1  "V_body"
  IC3/1 -> Demux1/1  "Omega_body"
  IC2/1 -> Demux3/1
  Bus Selector/1 -> Sum/2  "<Fgravity>"
  IC7/1 -> plantDataBus/10, Derivative/1  "alpha"
  envData1/1 -> Bus Selector1/1
  Bus Selector/2 -> Sum/3  "<Fground>"
  Bus Selector1/1 -> TransferFunction/1(In1)  "<windVelocity>"
  Sum2/1 -> "Incidence, Sideslip"/1("u, v, w")  "Vaero"
  Custom Variable Mass 6DOF (Euler Angles) (propio)/7(pdot,qdot,rdot) -> IC/1  "dOmega_body"
  Custom Variable Mass 6DOF (Euler Angles) (propio)/8(Ab) -> IC1/1  "Accel_body"
  IC8/1 -> Derivative1/1, plantDataBus/11  "beta"
  Sum1/1 -> IC10/1
  Sum/1 -> IC9/1
  IC9/1 -> Custom Variable Mass 6DOF (Euler Angles) (propio)/1(Forces)  "Fxyz"
  IC10/1 -> Custom Variable Mass 6DOF (Euler Angles) (propio)/2(Moments)  "Mxyz"
  IC/1 -> TransferFunctions/1(In1)  "dOmega_body"
  IC1/1 -> TransferFunctions/2(In2)  "Accel_body"
  TransferFunctions/1(Out1) -> plantDataBus/8  "dOmega_body"
  TransferFunctions/2(Out2) -> plantDataBus/9  "Accel_body"
  IC11/1 -> plantDataBus/2  "V_ned"
  IC12/1 -> plantDataBus/3  "X_ned"
  Rate Limiter1/1 -> plantDataBus/13  "beta_dot"
  TransferFunction/1(Out1) -> Sum2/2  "windVelocity"
  Rate Limiter/1 -> plantDataBus/12  "alpha_dot"
  Aerodynamics/2(Mbody) -> Sum1/1  "Maero"
  Aerodynamics/1(Fbody) -> Sum/1  "Faero_body"
  Bus Selector/3 -> Sum1/2  "<Mground>"
  Propulsion/2(Total_Thrust_Moment) -> Sum1/3  "Mthrust"
  Derivative/1 -> Rate Limiter/1
  Derivative1/1 -> Rate Limiter1/1

== system mainV02_37/Pilot Commands ==
  Bus Creator : BusCreator  Inputs=9  OutDataTypeStr=Bus: CommandBus  NonVirtualBus=on
  Signal Builder : Subsystem  Tag=STV Subsys  LoadFcn=sigbuilder_block('load');  StartFcn=sigbuilder_block('start');  StopFcn=sigbuilder_block('stop');  ClipboardFcn=sigbuilder_block('clipboard');  mask(Sigbuilder block){tuvar=[0:10]}
      mask help: Simulink:masks:SigbuilderBlock_MD
      mask init:
      | if ~strcmp(get_param(bdroot(gcbh),'SimulationStatus'),'stopped') tuvar = sigbuilder_block('maskInit'); end
      settings: CopyFcn=sigbuilder_block('copy');  DeleteFcn=sigbuilder_block('delete');  ModelCloseFcn=sigbuilder_block('modelClose');  PreSaveFcn=sigbuilder_block('preSave');  PauseFcn=sigbuilder_block('pause');  ContinueFcn=sigbuilder_block('continue');  NameChangeFcn=sigbuilder_block('namechange');  OpenFcn=sigbuilder_block('open',[234 6 960 605.25 ]);  CloseFcn=sigbuilder_block('close');
      mask Display: plot(0, 0, 100, 100,[2, 2, 32, 32, 2], [68, 8, 8, 68, 68],[32, 2], [38, 38], [32, 19, 2],[53, 60, 44], [32, 17, 17, 2],[16, 16, 31, 31]);txt = getActiveGroup(gcbh);text(2, 100, txt,'verticalAlignment', 'top');
  PilotCmd : Outport  OutDataTypeStr=Bus: CommandBus
  wires:
  Bus Creator/1 -> PilotCmd/1
  Signal Builder/1(Roll) -> Bus Creator/1  "roll_cmd"
  Signal Builder/2(Pitch) -> Bus Creator/2  "pitch_cmd"
  Signal Builder/3(Yaw) -> Bus Creator/3  "yaw_cmd"
  Signal Builder/4(Altitude) -> Bus Creator/4  "altitude_cmd"
  Signal Builder/9(Throttle5) -> Bus Creator/9  "Throttle5_cmd"
  Signal Builder/8(Throttle4) -> Bus Creator/8  "Throttle4_cmd"
  Signal Builder/7(Throttle3) -> Bus Creator/7  "Throttle3_cmd"
  Signal Builder/6(Throttle2) -> Bus Creator/6  "Throttle2_cmd"
  Signal Builder/5(Throttle1) -> Bus Creator/5  "Throttle1_cmd"
